simulink model "Use_Switch_block"  (R2024a)
settings: Solver=VariableStepAuto  StartTime=0.0  StopTime=10.0  MaxStep=1e-4  RelTol=1e-3
settings Model: Creator=admin  LastModifiedBy=admin

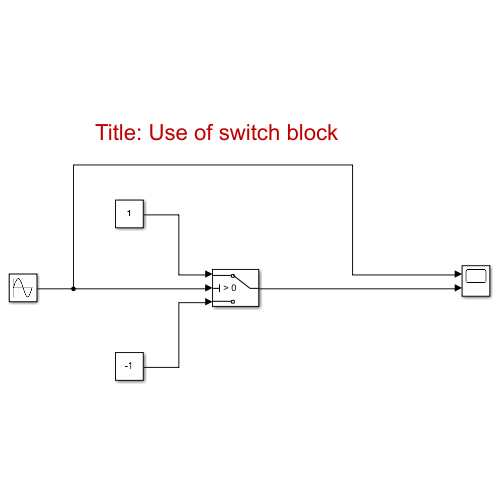
[thumbnail: Simulink's stored preview of the top-level diagram]
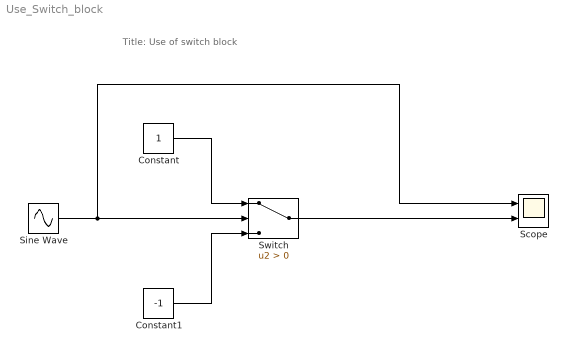
== system Use_Switch_block ==
  note: Title: Use of switch block
  Constant : Constant
  Constant1 : Constant  Value=-1
  Scope : Scope  NumInputPorts=2
  Sine Wave : Sin  SampleTime=0
  Switch : Switch  Criteria=u2 > Threshold  SaturateOnIntegerOverflow=off  InputSameDT=off
  wires:
  Sine Wave/1 -> Scope/1, Switch/2
  Constant/1 -> Switch/1
  Constant1/1 -> Switch/3
  Switch/1 -> Scope/2
